simulink model "state_fb_model"  (R2019a)
settings: Solver=ode4  StartTime=0.0  StopTime=10  FixedStep=0.001  RelTol=1e-3
undefined symbols (not defined in the file or in its folder): dat, K, whipple
settings Model: Creator=chris  LastModifiedBy=chris

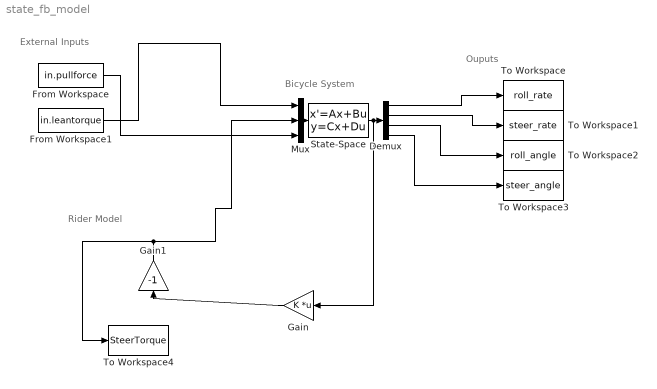
== system state_fb_model ==
  note: Bicycle System
  note: External Inputs
  note: Rider Model
  note: Ouputs
  Demux : Demux
  From Workspace : FromWorkspace  VariableName=in.pullforce  SampleTime=0
  From Workspace1 : FromWorkspace  VariableName=in.leantorque  SampleTime=0
  Gain : Gain  Gain=K  Multiplication=Matrix(K*u) (u vector)
  Gain1 : Gain  Gain=-1
  Mux : Mux  Inputs=3
  State-Space : StateSpace  A=[-whipple.M0 \ whipple.C1 * dat.v, -whipple.M0 \ (whipple.K0 + whipple.K2 * dat.v^2); eye(2), zeros(2)];  B=[whipple.M0 \ [eye(2), whipple.Hfw]; zeros(2, 3)]  C=eye(4)  D=zeros(4,3)  InitialCondition=0
  To Workspace : ToWorkspace  VariableName=roll_rate  SampleTime=-1
  To Workspace1 : ToWorkspace  VariableName=steer_rate  SampleTime=-1
  To Workspace2 : ToWorkspace  VariableName=roll_angle  SampleTime=-1
  To Workspace3 : ToWorkspace  VariableName=steer_angle  SampleTime=-1
  To Workspace4 : ToWorkspace  VariableName=SteerTorque  SampleTime=-1
  wires:
  Gain/1 -> Gain1/1
  Gain1/1 -> Mux/2, To Workspace4/1
  From Workspace/1 -> Mux/3
  Mux/1 -> State-Space/1
  Demux/1 -> To Workspace/1
  Demux/2 -> To Workspace1/1
  Demux/3 -> To Workspace2/1
  Demux/4 -> To Workspace3/1
  From Workspace1/1 -> Mux/1
  State-Space/1 -> Gain/1, Demux/1
